simulink model "position"  (R2022a)
settings: Solver=FixedStepAuto  StartTime=0.0  StopTime=inf  RelTol=1e-3
undefined symbols (not defined in the file or in its folder): X, Y, Z
libraries: robotlib x2
settings Model: Creator=alessandrini  LastModifiedBy=alessandrini
settings OptimizationCC: EnhancedBackFolding=on  PassReuseOutputArgsAs=Individual arguments  ZeroExternalMemoryAtStartup=off  ZeroInternalMemoryAtStartup=off  MaxStackSize=64  OptimizeBlockOrder=speed  DifferentSizesBufferReuse=on  OptimizationCustomize=off  EfficientTunableParamExpr=on
settings DebuggingCC: ParameterTunabilityLossMsg=error
settings HardwareCC: ProdBitPerPointer=32  ProdBitPerSizeT=32  ProdBitPerPtrDiffT=32  ProdLargestAtomicFloat=None  ProdIntDivRoundTo=Undefined  ProdEndianess=Unspecified  ProdWordSize=32  ProdHWDeviceType=Generic->Unspecified (assume 32-bit Generic)  UseEmbeddedCoderFeatures=off
settings SFSimCC: MATLABDynamicMemAlloc=off
settings RTWCC: SystemTargetFile=ert.tlc  HardwareBoard=Robot Operating System (ROS)  TLCOptions="-aInlineSetEventsForThisBaseRateFcn=TLC_FALSE -aSuppressMultiTaskScheduler=TLC_FALSE  -aRateBasedStepFcn=0"  TemplateMakefile=ert_default_tmf  Toolchain=Catkin  TargetLang=C++
settings CodeAppCC: ForceParamTrailComments=on  IgnoreCustomStorageClasses=off  OperatorAnnotations=on  SimulinkDataObjDesc=on  SFDataObjDesc=on  InsertBlockDesc=on
settings ERTTargetCC: SupportNonInlinedSFcns=on

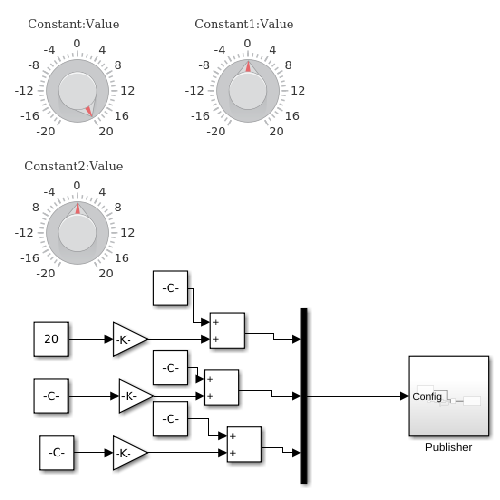
[thumbnail: Simulink's stored preview of the top-level diagram]
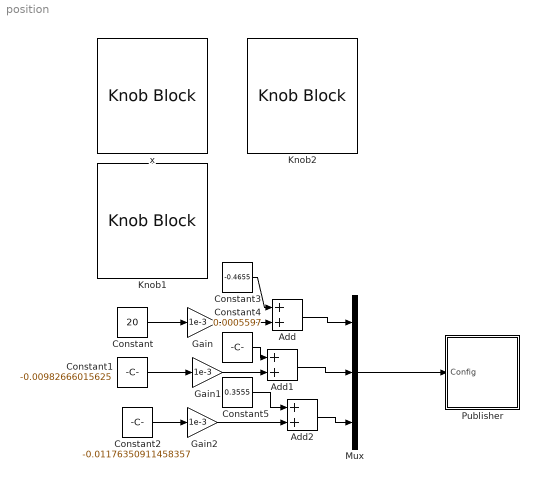
== system position ==
  Add : Sum
  Add1 : Sum
  Add2 : Sum
  Constant : Constant  Value=20
  Constant1 : Constant  Value=-0.00982666015625
  Constant2 : Constant  Value=-0.01176350911458357
  Constant3 : Constant  Value=-0.4655
  Constant4 : Constant  Value=0.0005597
  Constant5 : Constant  Value=0.3555
  Gain : Gain  Gain=1e-3
  Gain1 : Gain  Gain=1e-3
  Gain2 : Gain  Gain=1e-3
  Knob1 : KnobBlock  ScaleMin=-20  ScaleMax=20
  Knob2 : KnobBlock  ScaleMin=-20  ScaleMax=20
  Mux : Mux  Inputs=3
  Publisher : Subsystem
  x : KnobBlock  ScaleMin=-20  ScaleMax=20
  wires:
  Mux/1 -> Publisher/1(Config)
  Constant/1 -> Gain/1
  Constant1/1 -> Gain1/1
  Constant2/1 -> Gain2/1
  Gain/1 -> Add/2
  Add/1 -> Mux/1
  Constant3/1 -> Add/1
  Gain1/1 -> Add1/2
  Add1/1 -> Mux/2
  Constant4/1 -> Add1/1
  Gain2/1 -> Add2/2
  Add2/1 -> Mux/3
  Constant5/1 -> Add2/1

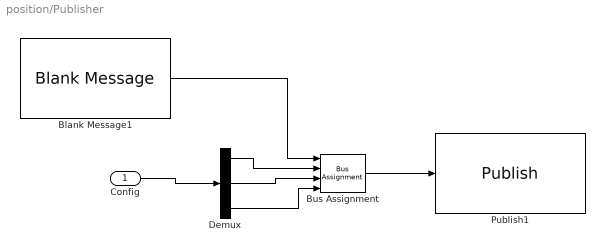
== system position/Publisher ==
  Config : Inport
  Blank Message1 : robotlib/Blank Message  messageClass=Message  entityType=geometry_msgs/Point  messageType=geometry_msgs/Point  SampleTime=0.02  legacyBusStruct=off
  Bus Assignment : BusAssignment  AssignedSignals=X,Y,Z
  Demux : Demux  Outputs=3
  Publish1 : robotlib/Publish  topicSource=Specify your own  topic=/Point/ref  messageType=geometry_msgs/Point  legacyBusStruct=off  messageQueueLength=1
  wires:
  Config/1 -> Demux/1
  Blank Message1/1 -> Bus Assignment/1
  Bus Assignment/1 -> Publish1/1
  Demux/1 -> Bus Assignment/2
  Demux/2 -> Bus Assignment/3
  Demux/3 -> Bus Assignment/4
